simulink model "pruebafmu"  (R2025a)
settings: Solver=FixedStepAuto  StartTime=0.0  StopTime=inf  FixedStep=0.001  RelTol=1e-3  EnableMultiTasking=on
libraries: px4Sensorslib x2, px4Peripheralslib x1
settings Model: PacingRate=0.790000  ExtModeTrigDuration=10  Creator=The MathWorks, Inc.  LastModifiedBy=aero
settings SolverCC: AlgebraicLoopSolver=TrustRegion  PositivePriorityOrder=on  AutoInsertRateTranBlk=on  MaxZcPerStep=1.0
settings OptimizationCC: EnhancedBackFolding=on  PassReuseOutputArgsAs=Individual arguments  MaxStackSize=64  OptimizeBlockOrder=speed  DifferentSizesBufferReuse=on  OptimizationCustomize=off  EfficientTunableParamExpr=on
settings DebuggingCC: ParameterPrecisionLossMsg=none  ParameterTunabilityLossMsg=error  UnconnectedInputMsg=warning  UnconnectedOutputMsg=warning  UnconnectedLineMsg=warning  SubsystemReferenceDiagnosticForUnitTest=warning  ArithmeticOperatorsInVariantConditions=warning
settings HardwareCC: ProdBitPerPointer=32.0  ProdBitPerSizeT=32.0  ProdBitPerPtrDiffT=32.0  ProdLargestAtomicInteger=Long  ProdLargestAtomicFloat=Double  ProdWordSize=32.0  ProdLongLongMode=on  ProdHWDeviceType=ARM Compatible->ARM Cortex
settings ModelReferenceCC: EnableRefExpFcnMdlSchedulingChecks=on
settings SFSimCC: MATLABDynamicMemAlloc=off  SimTargetLang=C++  SimDLTargetLibrary=mkl-dnn
settings RTWCC: SystemTargetFile=ert.tlc  HardwareBoard=PX4 Pixhawk 6c  TLCOptions="-aInlineSetEventsForThisBaseRateFcn=TLC_FALSE -aSuppressMultiTaskScheduler=TLC_FALSE  -aRateBasedStepFcn=0"  TemplateMakefile=ert_default_tmf  GenerateReport=on  Toolchain=GNU Tools for PX4 Autopilots  IncludeHyperlinkInReport=on  LaunchReport=on  TargetLang=C++  GenerateTraceInfo=on  GenerateTraceReport=on  GenerateTraceReportSl=on  GenerateTraceReportSf=on  GenerateTraceReportEml=on  GPUComputeCapability=3.5  DLArmComputeVersion=19.05  Description=Embedded Coder
settings CodeAppCC: ForceParamTrailComments=on  IgnoreCustomStorageClasses=off  OperatorAnnotations=on  SimulinkDataObjDesc=on  SFDataObjDesc=on  InsertBlockDesc=on
settings ERTTargetCC: ExtModeTransport=3.0  ExtModeStaticAllocSize=1024.0  InlinedParameterPlacement=Hierarchical

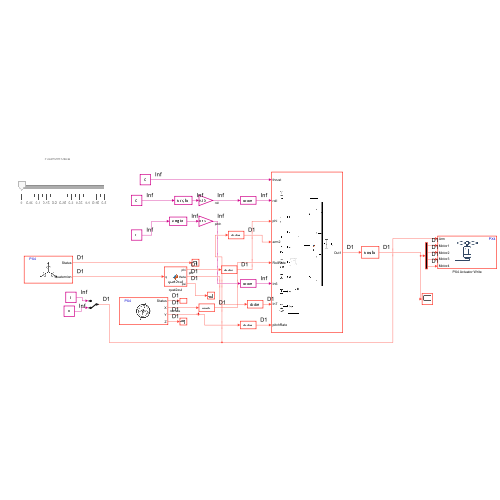
[thumbnail: Simulink's stored preview of the top-level diagram]
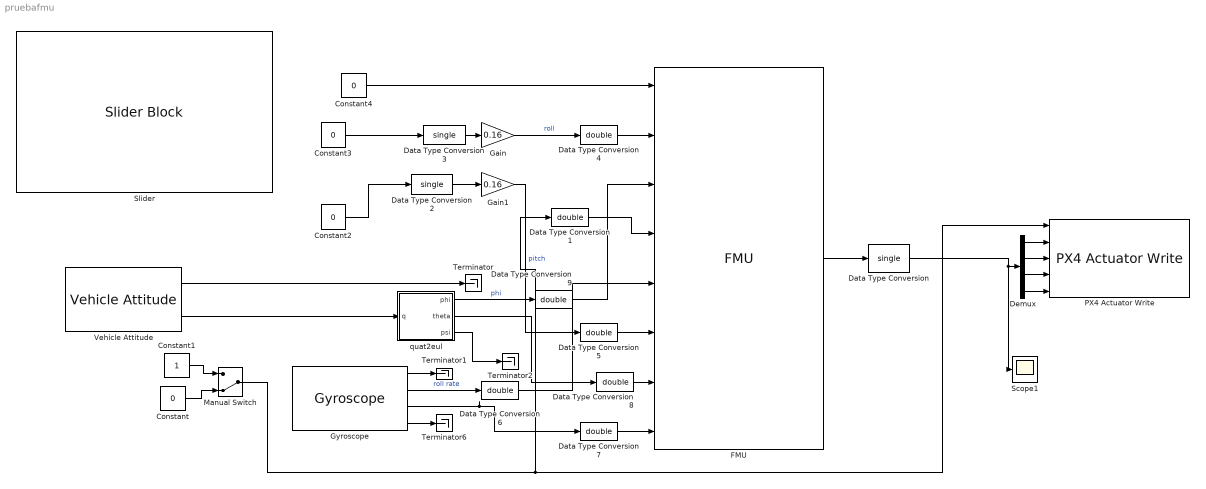
== system pruebafmu ==
  Constant : Constant  Value=0  OutDataTypeStr=boolean
  Constant1 : Constant  OutDataTypeStr=boolean
  Constant2 : Constant  Value=0
  Constant3 : Constant  Value=0
  Constant4 : Constant  Value=0
  Data Type Conversion : DataTypeConversion  OutDataTypeStr=single  SaturateOnIntegerOverflow=off  RndMeth=Floor
  Data Type Conversion{1,4..9} (7 alike) : DataTypeConversion  OutDataTypeStr=double  SaturateOnIntegerOverflow=off  RndMeth=Floor
  Data Type Conversion2 : DataTypeConversion  OutDataTypeStr=single  SaturateOnIntegerOverflow=off  RndMeth=Floor
  Data Type Conversion3 : DataTypeConversion  OutDataTypeStr=single  SaturateOnIntegerOverflow=off  RndMeth=Floor
  Demux : Demux
  FMU : FMU  FMUName=pruebafmu2.fmu  FMUMode=CoSimulation  FMUCreateBusObject=off  FMUInitializeEnumObject=off
      mask Type: pruebafmu2 [Co-Simulation, v2.0]
      mask Display:
      | if (exist([Simulink.fileGenControl('get','CacheFolder') '\slprj\_fmu\f2ec0e234a2d00d638c54fa383704903\pruebafmu2\model.png'],'file'))
      |     image([Simulink.fileGenControl('get','CacheFolder') '\slprj\_fmu\f2ec0e234a2d00d638c54fa383704903\pruebafmu2\model.png']);
      | else
      |     disp('pruebafmu2');
      | end
      | port_label('output',1,'Out1');
      | port_label('input',1,'thrust');
      | port_label('input',2,'roll');
      | port_label('input',3,'phi');
      | port_label('input',4,'arm2');
      | port_label('input',5,'RollRate');
      | port_label('input',6,'In6');
      | port_label('input',7,'In7');
      | port_label('input',8,'pitchRate');
  Gain : Gain  Gain=0.16
  Gain1 : Gain  Gain=0.16
  Gyroscope : px4Sensorslib/Gyroscope  uorbTimeStamp=off  BlockingMode=off  BlockTimeout=1e-3  sampleTime=0.001
  Manual Switch : ManualSwitch  CurrentSetting=0
  PX4 Actuator Write : px4Peripheralslib/PX4 Actuator Write  Motor1Enable=on  Motor2Enable=on  Motor3Enable=on  Motor4Enable=on  Motor5Enable=off  Motor6Enable=off  Motor7Enable=off  Motor8Enable=off  Motor9Enable=off  Motor10Enable=off  Motor11Enable=off  Motor12Enable=off  IsMotorArray=off  Servo1Enable=off  Servo2Enable=off  Servo3Enable=off  Servo4Enable=off  Servo5Enable=off  Servo6Enable=off  Servo7Enable=off  Servo8Enable=off  IsServoArray=off
  Scope1 : Scope
      settings: ActiveDisplayYMinimum=0.37234214547850747  ActiveDisplayYMaximum=0.42208466280379647  DataLoggingVariableName=ScopeData3
  Slider : SliderBlock  ScaleMax=0.5
  Terminator{,1..2,6} (4 alike) : Terminator
  Vehicle Attitude : px4Sensorslib/Vehicle Attitude  rollRate=off  pitchRate=off  yawRate=off  quaternion=on  uorbTimeStamp=off  BlockingMode=off  BlockTimeout=0.001  sampleTime=0.001
  quat2eul : MATLAB Function  TreatAsAtomicUnit=on
  wires:
  Manual Switch/1 -> Data Type Conversion1/1, PX4 Actuator Write/1
  Vehicle Attitude/1 -> Terminator/1
  Gyroscope/1 -> Terminator1/1
  Gain/1 -> Data Type Conversion4/1  "roll"
  Data Type Conversion/1 -> Scope1/1, Demux/1
  Demux/1 -> PX4 Actuator Write/2
  Demux/2 -> PX4 Actuator Write/3
  Demux/3 -> PX4 Actuator Write/4
  Demux/4 -> PX4 Actuator Write/5
  Constant/1 -> Manual Switch/2
  Constant1/1 -> Manual Switch/1
  Gyroscope/2 -> Data Type Conversion6/1  "roll rate"
  Gyroscope/4 -> Terminator6/1
  Gyroscope/3 -> Data Type Conversion7/1
  Gain1/1 -> Data Type Conversion5/1  "pitch"
  Data Type Conversion3/1 -> Gain/1
  Data Type Conversion2/1 -> Gain1/1
  Constant2/1 -> Data Type Conversion2/1
  Constant3/1 -> Data Type Conversion3/1
  Vehicle Attitude/2 -> quat2eul/1(q)
  quat2eul/2(theta) -> Data Type Conversion8/1
  quat2eul/1(phi) -> Data Type Conversion9/1  "phi"
  quat2eul/3(psi) -> Terminator2/1
  Constant4/1 -> FMU/1
  FMU/1 -> Data Type Conversion/1
  Data Type Conversion1/1 -> FMU/4
  Data Type Conversion4/1 -> FMU/2
  Data Type Conversion5/1 -> FMU/6
  Data Type Conversion6/1 -> FMU/5
  Data Type Conversion7/1 -> FMU/8
  Data Type Conversion8/1 -> FMU/7
  Data Type Conversion9/1 -> FMU/3

== matlab function pruebafmu/quat2eul ==
  data: q input; phi output; theta output; psi output
function [phi,theta,psi] = quat2eul(q)

% Quaternion conversion to Euler angles based on the PX4 Firmware v1.10.2
% release.

phi = atan2(2*(q(1)*q(2) + q(3)* q(4)), q(1)^2 - q(2)^2 - q(3)^2 + q(4)^2);
theta = asin(-2*(q(2)*q(4) - q(1)*q(3)));
psi = atan2(2*(q(2)*q(3) + q(1)* q(4)), q(1)^2 + q(2)^2 - q(3)^2 - q(4)^2);
end
